simulink model "TiribaFlightControl"  (Simulink 7.6)
settings: Solver=ode45  StartTime=0.0  StopTime=10.0  RelTol=1e-3
Description:
  | <HiP-HOPS_Model_Parameters><ToolVersion><Name>Matlab</Name><Number>7.11.0.584 </Number></ToolVersion><RiskTime>10000</RiskTime><OptimisationParams><MaxGenerations>100</MaxGenerations></OptimisationParams><Hazards><Hazard><Name>No_Pilot_Commands</Name><Description></Description><SafetyRequirement>4</SafetyRequirement><Causes><Cause><Probability></Probability><FailureLogic>Omission-PWMDecoder.FlightControls AND Omission-FailSafeController.FilteredControls</FailureLogic></Cause></Causes></Hazard><Hazard><Name>Value_Pilot_Commands</Name><Description></Description><SafetyRequirement>4</SafetyRequirement><Causes><Cause><Probability></Probability><FailureLogic>Value-PWMDecoder.FlightControls AND Value-FailSafeController.FilteredControls</FailureLogic></Cause></Causes></Hazard></Hazards><AdvancedParameters></AdvancedParameters></HiP-HOPS_Model_Parameters>
settings Model: Creator=Andre  LastModifiedBy=Andre

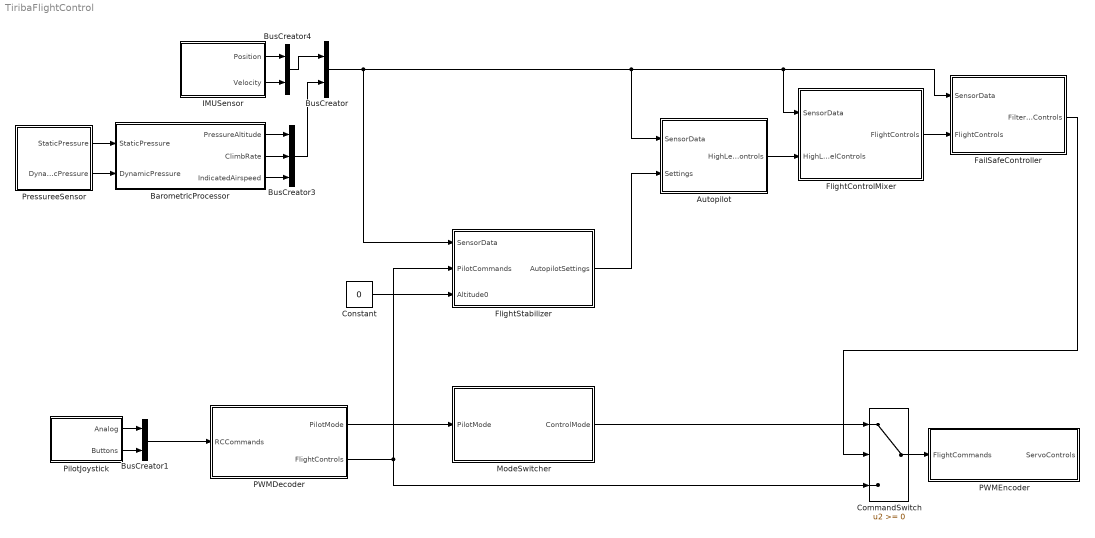
== system TiribaFlightControl ==
  Autopilot : Subsystem
  BarometricProcessor : Subsystem
  BusCreator : BusCreator  Inputs=2
  BusCreator1 : BusCreator  Inputs=2
  BusCreator3 : BusCreator  Inputs=3
  BusCreator4 : BusCreator  Inputs=2
  CommandSwitch : Switch
  Constant : Constant  Value=0
  FailSafeController : Subsystem
  FlightControlMixer : Subsystem
  FlightStabilizer : Subsystem
  IMUSensor : Subsystem
  ModeSwitcher : Subsystem
  PWMDecoder : Subsystem
  PWMEncoder : Subsystem
  PilotJoystick : Subsystem
  PressureeSensor : Subsystem
  wires:
  CommandSwitch/1 -> PWMEncoder/1(FlightCommands)
  FailSafeController/1(FilteredControls) -> CommandSwitch/2
  FlightControlMixer/1(FlightControls) -> FailSafeController/2(FlightControls)
  BusCreator/1 -> FlightControlMixer/1(SensorData), FailSafeController/1(SensorData), Autopilot/1(SensorData), FlightStabilizer/1(SensorData)
  Autopilot/1(HighLevelControls) -> FlightControlMixer/2(HighLevelControls)
  FlightStabilizer/1(AutopilotSettings) -> Autopilot/2(Settings)
  Constant/1 -> FlightStabilizer/3(Altitude0)
  PWMDecoder/1(PilotMode) -> ModeSwitcher/1(PilotMode)
  PWMDecoder/2(FlightControls) -> CommandSwitch/3, FlightStabilizer/2(PilotCommands)
  ModeSwitcher/1(ControlMode) -> CommandSwitch/1
  PilotJoystick/1(Analog) -> BusCreator1/1
  PilotJoystick/2(Buttons) -> BusCreator1/2
  BusCreator1/1 -> PWMDecoder/1(RCCommands)
  IMUSensor/1(Position) -> BusCreator4/1
  IMUSensor/2(Velocity) -> BusCreator4/2
  BarometricProcessor/1(PressureAltitude) -> BusCreator3/1
  BarometricProcessor/2(ClimbRate) -> BusCreator3/2
  BarometricProcessor/3(IndicatedAirspeed) -> BusCreator3/3
  PressureeSensor/1(StaticPressure) -> BarometricProcessor/1(StaticPressure)
  PressureeSensor/2(DynamicPressure) -> BarometricProcessor/2(DynamicPressure)
  BusCreator4/1 -> BusCreator/1
  BusCreator3/1 -> BusCreator/2

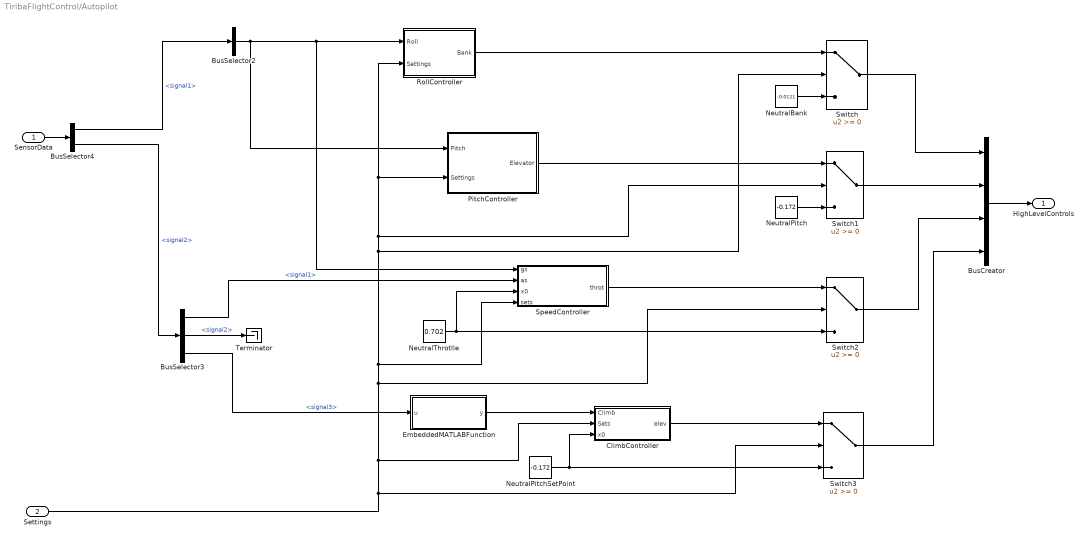
== system TiribaFlightControl/Autopilot ==
  SensorData : Inport
  Settings : Inport  Port=2
  BusCreator : BusCreator
  BusSelector2 : BusSelector  OutputSignals=signal2  OutputAsBus=on
  BusSelector3 : BusSelector  OutputSignals=signal1,signal2,signal3
  BusSelector4 : BusSelector  OutputSignals=signal1,signal2
  ClimbController : Subsystem
  EmbeddedMATLABFunction : Subsystem
  NeutralBank : Constant  Value=-0.0121
  NeutralPitch : Constant  Value=-0.172
  NeutralPitchSetPoint : Constant  Value=-0.172
  NeutralThrotlle : Constant  Value=0.702
  PitchController : Subsystem
  RollController : Subsystem
  SpeedController : Subsystem
  Switch{,1..3} (4 alike) : Switch
  Terminator : Terminator
  HighLevelControls : Outport
  wires:
  Settings/1 -> Switch/2, RollController/2(Settings), PitchController/2(Settings), Switch1/2, SpeedController/4(sets), Switch2/2, ClimbController/2(Sets), Switch3/2
  SensorData/1 -> BusSelector4/1
  BusSelector2/1 -> PitchController/1(Pitch), RollController/1(Roll), SpeedController/1(gs)
  RollController/1(Bank) -> Switch/1
  NeutralBank/1 -> Switch/3
  PitchController/1(Elevator) -> Switch1/1
  NeutralPitch/1 -> Switch1/3
  BusSelector3/2 -> Terminator/1  "<signal2>"
  BusSelector3/1 -> SpeedController/2(as)  "<signal1>"
  SpeedController/1(throt) -> Switch2/1
  NeutralThrotlle/1 -> SpeedController/3(x0), Switch2/3
  BusSelector3/3 -> EmbeddedMATLABFunction/1(u)  "<signal3>"
  NeutralPitchSetPoint/1 -> ClimbController/3(x0), Switch3/3
  ClimbController/1(elev) -> Switch3/1
  EmbeddedMATLABFunction/1(y) -> ClimbController/1(Climb)
  Switch/1 -> BusCreator/1
  Switch1/1 -> BusCreator/2
  Switch2/1 -> BusCreator/3
  Switch3/1 -> BusCreator/4
  BusCreator/1 -> HighLevelControls/1
  BusSelector4/1 -> BusSelector2/1  "<signal1>"
  BusSelector4/2 -> BusSelector3/1  "<signal2>"

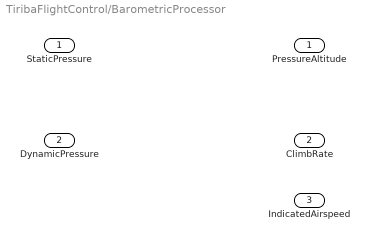
== system TiribaFlightControl/BarometricProcessor ==
  StaticPressure : Inport
  DynamicPressure : Inport  Port=2
  PressureAltitude : Outport
  ClimbRate : Outport  Port=2
  IndicatedAirspeed : Outport  Port=3

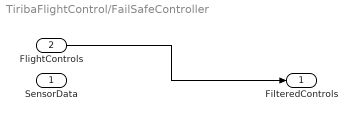
== system TiribaFlightControl/FailSafeController ==
  SensorData : Inport
  FlightControls : Inport  Port=2
  FilteredControls : Outport
  wires:
  FlightControls/1 -> FilteredControls/1

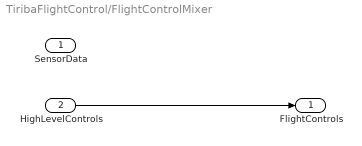
== system TiribaFlightControl/FlightControlMixer ==
  SensorData : Inport
  HighLevelControls : Inport  Port=2
  FlightControls : Outport
  wires:
  HighLevelControls/1 -> FlightControls/1

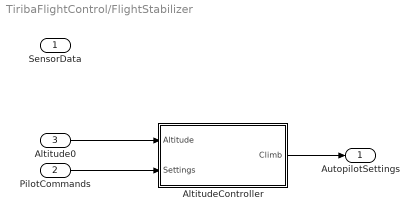
== system TiribaFlightControl/FlightStabilizer ==
  SensorData : Inport
  PilotCommands : Inport  Port=2
  Altitude0 : Inport  Port=3
  AltitudeController : Subsystem
  AutopilotSettings : Outport
  wires:
  PilotCommands/1 -> AltitudeController/2(Settings)
  Altitude0/1 -> AltitudeController/1(Altitude)
  AltitudeController/1(Climb) -> AutopilotSettings/1

== system TiribaFlightControl/IMUSensor ==
  Position : Outport
  Velocity : Outport  Port=2

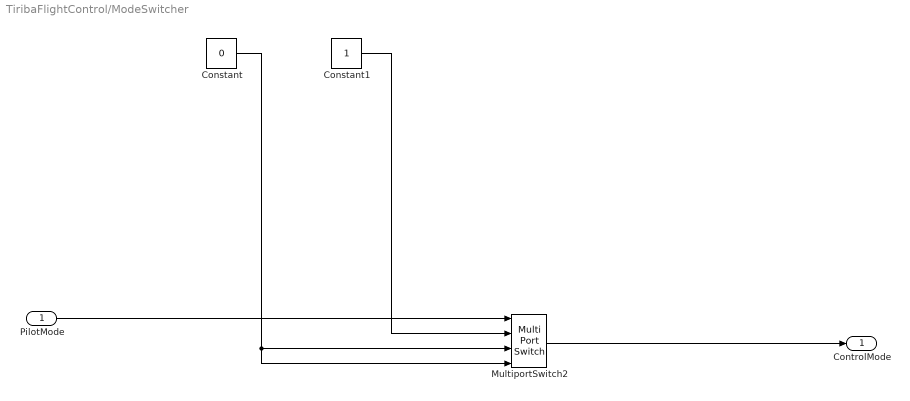
== system TiribaFlightControl/ModeSwitcher ==
  PilotMode : Inport
  Constant : Constant  Value=0
  Constant1 : Constant
  MultiportSwitch2 : MultiPortSwitch  zeroidx=off
  ControlMode : Outport
  wires:
  PilotMode/1 -> MultiportSwitch2/1
  MultiportSwitch2/1 -> ControlMode/1
  Constant/1 -> MultiportSwitch2/4, MultiportSwitch2/3
  Constant1/1 -> MultiportSwitch2/2

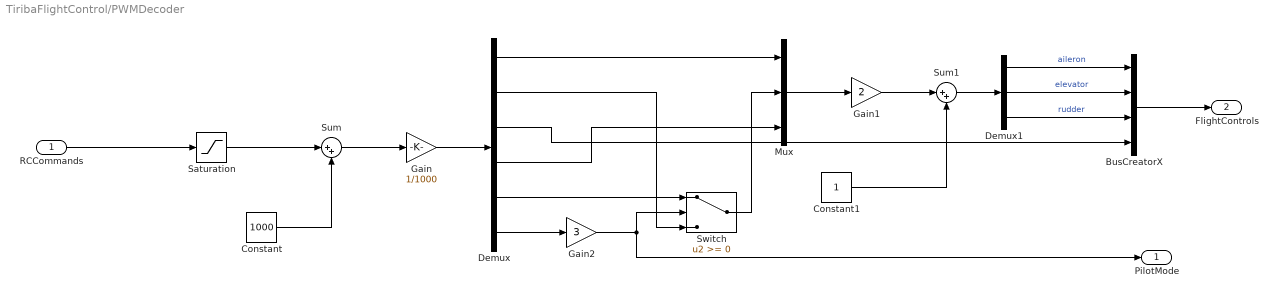
== system TiribaFlightControl/PWMDecoder ==
  RCCommands : Inport
  BusCreatorX : BusCreator
  Constant : Constant  Value=1000
  Constant1 : Constant
  Demux : Demux  Outputs=6
  Demux1 : Demux  Outputs=3
  Gain : Gain  Gain=1/1000
  Gain1 : Gain  Gain=2
  Gain2 : Gain  Gain=3
  Mux : Mux  Inputs=3
  Saturation : Saturate
  Sum : Sum  Inputs=|++
  Sum1 : Sum  Inputs=|++
  Switch : Switch
  PilotMode : Outport
  FlightControls : Outport  Port=2
  wires:
  RCCommands/1 -> Saturation/1
  Saturation/1 -> Sum/1
  Constant/1 -> Sum/2
  Sum/1 -> Gain/1
  Gain/1 -> Demux/1
  Demux/1 -> Mux/1
  Demux/4 -> Mux/3
  Mux/1 -> Gain1/1
  Gain1/1 -> Sum1/1
  Constant1/1 -> Sum1/2
  Sum1/1 -> Demux1/1
  Demux/3 -> BusCreatorX/4
  Demux1/3 -> BusCreatorX/3  "rudder"
  Demux1/2 -> BusCreatorX/2  "elevator"
  Demux1/1 -> BusCreatorX/1  "aileron"
  BusCreatorX/1 -> FlightControls/1
  Gain2/1 -> Switch/2, PilotMode/1
  Demux/2 -> Switch/3
  Demux/6 -> Gain2/1
  Demux/5 -> Switch/1
  Switch/1 -> Mux/2

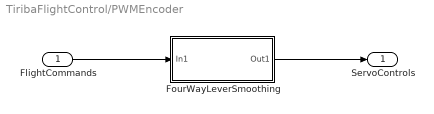
== system TiribaFlightControl/PWMEncoder ==
  FlightCommands : Inport
  FourWayLeverSmoothing : Subsystem
  ServoControls : Outport
  wires:
  FlightCommands/1 -> FourWayLeverSmoothing/1(In1)
  FourWayLeverSmoothing/1(Out1) -> ServoControls/1

== system TiribaFlightControl/PilotJoystick ==
  Analog : Outport
  Buttons : Outport  Port=2

== system TiribaFlightControl/PressureeSensor ==
  StaticPressure : Outport
  DynamicPressure : Outport  Port=2

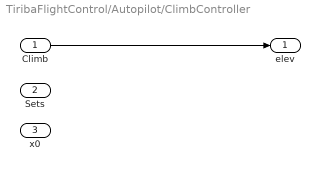
== system TiribaFlightControl/Autopilot/ClimbController ==
  Climb : Inport
  Sets : Inport  Port=2
  x0 : Inport  Port=3
  elev : Outport
  wires:
  Climb/1 -> elev/1

== system TiribaFlightControl/Autopilot/EmbeddedMATLABFunction ==
  u : Inport
  y : Outport
  wires:
  u/1 -> y/1

== system TiribaFlightControl/Autopilot/PitchController ==
  Pitch : Inport
  Settings : Inport  Port=2
  Elevator : Outport
  wires:
  Settings/1 -> Elevator/1

== system TiribaFlightControl/Autopilot/RollController ==
  Roll : Inport
  Settings : Inport  Port=2
  Bank : Outport
  wires:
  Roll/1 -> Bank/1

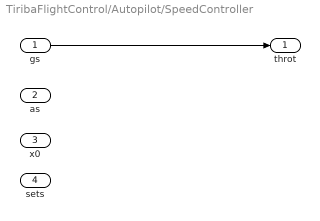
== system TiribaFlightControl/Autopilot/SpeedController ==
  gs : Inport
  as : Inport  Port=2
  x0 : Inport  Port=3
  sets : Inport  Port=4
  throt : Outport
  wires:
  gs/1 -> throt/1

== system TiribaFlightControl/FlightStabilizer/AltitudeController ==
  Altitude : Inport
  Settings : Inport  Port=2
  Climb : Outport
  wires:
  Altitude/1 -> Climb/1

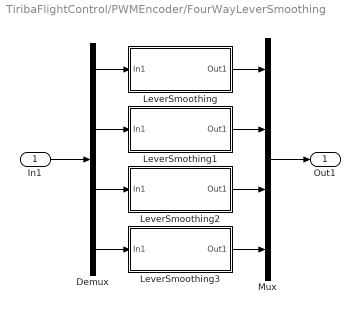
== system TiribaFlightControl/PWMEncoder/FourWayLeverSmoothing ==
  In1 : Inport
  Demux : Demux
  LeverSmoothing : Subsystem
  LeverSmoothing2 : Subsystem
  LeverSmoothing3 : Subsystem
  LeverSmothing1 : Subsystem
  Mux : Mux
  Out1 : Outport
  wires:
  In1/1 -> Demux/1
  Demux/1 -> LeverSmoothing/1(In1)
  LeverSmoothing/1(Out1) -> Mux/1
  Demux/2 -> LeverSmothing1/1(In1)
  LeverSmothing1/1(Out1) -> Mux/2
  Demux/3 -> LeverSmoothing2/1(In1)
  LeverSmoothing2/1(Out1) -> Mux/3
  Demux/4 -> LeverSmoothing3/1(In1)
  LeverSmoothing3/1(Out1) -> Mux/4
  Mux/1 -> Out1/1

== system TiribaFlightControl/PWMEncoder/FourWayLeverSmoothing/LeverSmoothing ==
  In1 : Inport
  Out1 : Outport
  wires:
  In1/1 -> Out1/1

== system TiribaFlightControl/PWMEncoder/FourWayLeverSmoothing/LeverSmoothing2 ==
  In1 : Inport
  Out1 : Outport
  wires:
  In1/1 -> Out1/1

== system TiribaFlightControl/PWMEncoder/FourWayLeverSmoothing/LeverSmoothing3 ==
  In1 : Inport
  Out1 : Outport
  wires:
  In1/1 -> Out1/1

== system TiribaFlightControl/PWMEncoder/FourWayLeverSmoothing/LeverSmothing1 ==
  In1 : Inport
  Out1 : Outport
  wires:
  In1/1 -> Out1/1
